simulink model "b_2x_8a_r308d"  (Simulink 6.2)
settings: Solver=ode45  StartTime=0.0  StopTime=1030.0  RelTol=1e-3
undefined symbols (not defined in the file): ant_bits, BEE2_usr, blockCountBits, blockRowBits, cmult_4bit_em
libraries: xbsIndex_r3 x3300, xps_library x102, casper_library x97
(part 14 of 22)

== system b_2x_8a_r308d/win_x_engine1/auto_tap/dual_pol_cmac/cmac1 ==
  a+bi : Inport  Port=1  LatchInput=off
  c+di : Inport  Port=2  LatchInput=off
  acc_in : Inport  Port=3  LatchInput=off
  sync : Inport  Port=4  LatchInput=off
  valid_in : Inport  Port=5  LatchInput=off
  Constant1 : xbsIndex_r3/Constant  const=0  equ=P=C  arith_type=Unsigned  n_bits=bit_growth  bin_pt=0  opselect=C  inp2=PCIN>>17  opr=+  inp1=P  carry=CIN  iostate=0  explicit_period=off  period=1  dbl_ovrd=off
  Constant2 : xbsIndex_r3/Constant  const=0  equ=P=C  arith_type=Unsigned  n_bits=1  bin_pt=0  opselect=C  inp2=PCIN>>17  opr=+  inp1=P  carry=CIN  iostate=0  explicit_period=off  period=1  dbl_ovrd=off
  Counter : xbsIndex_r3/Counter  cnt_type=Count Limited  n_bits=bit_growth  bin_pt=0  arith_type=Unsigned  start_count=0  cnt_to=acc_len - 1  cnt_by_val=1  operation=Up  explicit_period=off  period=1  load_pin=off  rst=on  en=off  dbl_ovrd=off  show_param=off  use_rpm=on  gen_core=off
      settings: xl_area=[0, 0, 0, 0, 0, 0, 0]
  Delay : xbsIndex_r3/Delay  latency=add_latency + mult_latency - 1  reg_retiming=off  explicit_period=off  period=1  en=off  accept_only_valid=off  init_zero=on  dbl_ovrd=off  show_param=off
      settings: xl_area=[0, 0, 0, 0, 0, 0, 0]
  Relational : xbsIndex_r3/Relational  mode=a=b  latency=1  explicit_period=off  period=1  en=off  dbl_ovrd=off  show_param=off
      settings: xl_area=[0, 0, 0, 0, 0, 0, 0]
  Terminator : Terminator
  acc : Subsystem
  acc1 : Subsystem
  c_to_ri : Subsystem
  c_to_ri1 : Subsystem
  c_to_ri2 : Subsystem
  cmult* : Subsystem  BlockChoice=cmult_4bit_em*
      link override cmult_4bit_br*: mult_latency=mult_latency  add_latency=add_latency
      link override cmult_4bit_em*: mult_latency=mult_latency  add_latency=add_latency
      link override cmult_4bit_sl*: mult_latency=mult_latency  add_latency=add_latency
      settings: AttributesFormatString=%<BlockChoice>  TemplateBlock=casper_library/Multipliers/cmult*  MemberBlocks=cmult_4bit_br*,cmult_4bit_em*,cmult_4bit_sl*
      mask Type: cmult*
  ri_to_c : Subsystem
  acc_out : Outport
  valid_out : Outport  Port=2
  wires:
  valid_in/1 -> acc1/4(valid_in)
  acc1/2(valid_out) -> valid_out/1
  acc/2(valid_out) -> Terminator/1
  Constant2/1 -> acc/4(valid_in)
  Delay/1 -> Counter/1
  sync/1 -> Delay/1
  Constant1/1 -> Relational/2
  Counter/1 -> Relational/1
  Relational/1 -> acc1/1(rst), acc/1(rst)
  c_to_ri2/2(Out2) -> acc1/3(acc_in)
  c_to_ri2/1(Out1) -> acc/3(acc_in)
  ri_to_c/1(Out1) -> acc_out/1
  acc1/1(acc_out) -> ri_to_c/2(In2)
  acc/1(acc_out) -> ri_to_c/1(In1)
  acc_in/1 -> c_to_ri2/1(In1)
  c_to_ri1/2(Out2) -> cmult*/4(d)
  c_to_ri1/1(Out1) -> cmult*/3(c)
  c+di/1 -> c_to_ri1/1(In1)
  c_to_ri/2(Out2) -> cmult*/2(b)
  c_to_ri/1(Out1) -> cmult*/1(a)
  a+bi/1 -> c_to_ri/1(In1)
  cmult*/2(imag) -> acc1/2(din)
  cmult*/1(real) -> acc/2(din)

== system b_2x_8a_r308d/win_x_engine1/auto_tap/dual_pol_cmac/cmac2 ==
  a+bi : Inport  Port=1  LatchInput=off
  c+di : Inport  Port=2  LatchInput=off
  acc_in : Inport  Port=3  LatchInput=off
  sync : Inport  Port=4  LatchInput=off
  valid_in : Inport  Port=5  LatchInput=off
  Constant1 : xbsIndex_r3/Constant  const=0  equ=P=C  arith_type=Unsigned  n_bits=bit_growth  bin_pt=0  opselect=C  inp2=PCIN>>17  opr=+  inp1=P  carry=CIN  iostate=0  explicit_period=off  period=1  dbl_ovrd=off
  Constant2 : xbsIndex_r3/Constant  const=0  equ=P=C  arith_type=Unsigned  n_bits=1  bin_pt=0  opselect=C  inp2=PCIN>>17  opr=+  inp1=P  carry=CIN  iostate=0  explicit_period=off  period=1  dbl_ovrd=off
  Counter : xbsIndex_r3/Counter  cnt_type=Count Limited  n_bits=bit_growth  bin_pt=0  arith_type=Unsigned  start_count=0  cnt_to=acc_len - 1  cnt_by_val=1  operation=Up  explicit_period=off  period=1  load_pin=off  rst=on  en=off  dbl_ovrd=off  show_param=off  use_rpm=on  gen_core=off
      settings: xl_area=[0, 0, 0, 0, 0, 0, 0]
  Delay : xbsIndex_r3/Delay  latency=add_latency + mult_latency - 1  reg_retiming=off  explicit_period=off  period=1  en=off  accept_only_valid=off  init_zero=on  dbl_ovrd=off  show_param=off
      settings: xl_area=[0, 0, 0, 0, 0, 0, 0]
  Relational : xbsIndex_r3/Relational  mode=a=b  latency=1  explicit_period=off  period=1  en=off  dbl_ovrd=off  show_param=off
      settings: xl_area=[0, 0, 0, 0, 0, 0, 0]
  Terminator : Terminator
  acc : Subsystem
  acc1 : Subsystem
  c_to_ri : Subsystem
  c_to_ri1 : Subsystem
  c_to_ri2 : Subsystem
  cmult* : Subsystem  BlockChoice=cmult_4bit_em*
      link override cmult_4bit_br*: mult_latency=mult_latency  add_latency=add_latency
      link override cmult_4bit_em*: mult_latency=mult_latency  add_latency=add_latency
      link override cmult_4bit_sl*: mult_latency=mult_latency  add_latency=add_latency
      settings: AttributesFormatString=%<BlockChoice>  TemplateBlock=casper_library/Multipliers/cmult*  MemberBlocks=cmult_4bit_br*,cmult_4bit_em*,cmult_4bit_sl*
      mask Type: cmult*
  ri_to_c : Subsystem
  acc_out : Outport
  valid_out : Outport  Port=2
  wires:
  cmult*/1(real) -> acc/2(din)
  cmult*/2(imag) -> acc1/2(din)
  a+bi/1 -> c_to_ri/1(In1)
  c_to_ri/1(Out1) -> cmult*/1(a)
  c_to_ri/2(Out2) -> cmult*/2(b)
  c+di/1 -> c_to_ri1/1(In1)
  c_to_ri1/1(Out1) -> cmult*/3(c)
  c_to_ri1/2(Out2) -> cmult*/4(d)
  acc_in/1 -> c_to_ri2/1(In1)
  acc/1(acc_out) -> ri_to_c/1(In1)
  acc1/1(acc_out) -> ri_to_c/2(In2)
  ri_to_c/1(Out1) -> acc_out/1
  c_to_ri2/1(Out1) -> acc/3(acc_in)
  c_to_ri2/2(Out2) -> acc1/3(acc_in)
  Relational/1 -> acc/1(rst), acc1/1(rst)
  Counter/1 -> Relational/1
  Constant1/1 -> Relational/2
  sync/1 -> Delay/1
  Delay/1 -> Counter/1
  Constant2/1 -> acc/4(valid_in)
  acc/2(valid_out) -> Terminator/1
  acc1/2(valid_out) -> valid_out/1
  valid_in/1 -> acc1/4(valid_in)

== system b_2x_8a_r308d/win_x_engine1/auto_tap/dual_pol_cmac/cmac3 ==
  a+bi : Inport  Port=1  LatchInput=off
  c+di : Inport  Port=2  LatchInput=off
  acc_in : Inport  Port=3  LatchInput=off
  sync : Inport  Port=4  LatchInput=off
  valid_in : Inport  Port=5  LatchInput=off
  Constant1 : xbsIndex_r3/Constant  const=0  equ=P=C  arith_type=Unsigned  n_bits=bit_growth  bin_pt=0  opselect=C  inp2=PCIN>>17  opr=+  inp1=P  carry=CIN  iostate=0  explicit_period=off  period=1  dbl_ovrd=off
  Constant2 : xbsIndex_r3/Constant  const=0  equ=P=C  arith_type=Unsigned  n_bits=1  bin_pt=0  opselect=C  inp2=PCIN>>17  opr=+  inp1=P  carry=CIN  iostate=0  explicit_period=off  period=1  dbl_ovrd=off
  Counter : xbsIndex_r3/Counter  cnt_type=Count Limited  n_bits=bit_growth  bin_pt=0  arith_type=Unsigned  start_count=0  cnt_to=acc_len - 1  cnt_by_val=1  operation=Up  explicit_period=off  period=1  load_pin=off  rst=on  en=off  dbl_ovrd=off  show_param=off  use_rpm=on  gen_core=off
      settings: xl_area=[0, 0, 0, 0, 0, 0, 0]
  Delay : xbsIndex_r3/Delay  latency=add_latency + mult_latency - 1  reg_retiming=off  explicit_period=off  period=1  en=off  accept_only_valid=off  init_zero=on  dbl_ovrd=off  show_param=off
      settings: xl_area=[0, 0, 0, 0, 0, 0, 0]
  Relational : xbsIndex_r3/Relational  mode=a=b  latency=1  explicit_period=off  period=1  en=off  dbl_ovrd=off  show_param=off
      settings: xl_area=[0, 0, 0, 0, 0, 0, 0]
  Terminator : Terminator
  acc : Subsystem
  acc1 : Subsystem
  c_to_ri : Subsystem
  c_to_ri1 : Subsystem
  c_to_ri2 : Subsystem
  cmult* : Subsystem  BlockChoice=cmult_4bit_em*
      link override cmult_4bit_br*: mult_latency=mult_latency  add_latency=add_latency
      link override cmult_4bit_em*: mult_latency=mult_latency  add_latency=add_latency
      link override cmult_4bit_sl*: mult_latency=mult_latency  add_latency=add_latency
      settings: AttributesFormatString=%<BlockChoice>  TemplateBlock=casper_library/Multipliers/cmult*  MemberBlocks=cmult_4bit_br*,cmult_4bit_em*,cmult_4bit_sl*
      mask Type: cmult*
  ri_to_c : Subsystem
  acc_out : Outport
  valid_out : Outport  Port=2
  wires:
  cmult*/1(real) -> acc/2(din)
  cmult*/2(imag) -> acc1/2(din)
  a+bi/1 -> c_to_ri/1(In1)
  c_to_ri/1(Out1) -> cmult*/1(a)
  c_to_ri/2(Out2) -> cmult*/2(b)
  c+di/1 -> c_to_ri1/1(In1)
  c_to_ri1/1(Out1) -> cmult*/3(c)
  c_to_ri1/2(Out2) -> cmult*/4(d)
  acc_in/1 -> c_to_ri2/1(In1)
  acc/1(acc_out) -> ri_to_c/1(In1)
  acc1/1(acc_out) -> ri_to_c/2(In2)
  ri_to_c/1(Out1) -> acc_out/1
  c_to_ri2/1(Out1) -> acc/3(acc_in)
  c_to_ri2/2(Out2) -> acc1/3(acc_in)
  Relational/1 -> acc/1(rst), acc1/1(rst)
  Counter/1 -> Relational/1
  Constant1/1 -> Relational/2
  sync/1 -> Delay/1
  Delay/1 -> Counter/1
  Constant2/1 -> acc/4(valid_in)
  acc/2(valid_out) -> Terminator/1
  acc1/2(valid_out) -> valid_out/1
  valid_in/1 -> acc1/4(valid_in)

== system b_2x_8a_r308d/win_x_engine1/auto_tap/dual_pol_cmac/cmac4 ==
  a+bi : Inport  Port=1  LatchInput=off
  c+di : Inport  Port=2  LatchInput=off
  acc_in : Inport  Port=3  LatchInput=off
  sync : Inport  Port=4  LatchInput=off
  valid_in : Inport  Port=5  LatchInput=off
  Constant1 : xbsIndex_r3/Constant  const=0  equ=P=C  arith_type=Unsigned  n_bits=bit_growth  bin_pt=0  opselect=C  inp2=PCIN>>17  opr=+  inp1=P  carry=CIN  iostate=0  explicit_period=off  period=1  dbl_ovrd=off
  Constant2 : xbsIndex_r3/Constant  const=0  equ=P=C  arith_type=Unsigned  n_bits=1  bin_pt=0  opselect=C  inp2=PCIN>>17  opr=+  inp1=P  carry=CIN  iostate=0  explicit_period=off  period=1  dbl_ovrd=off
  Counter : xbsIndex_r3/Counter  cnt_type=Count Limited  n_bits=bit_growth  bin_pt=0  arith_type=Unsigned  start_count=0  cnt_to=acc_len - 1  cnt_by_val=1  operation=Up  explicit_period=off  period=1  load_pin=off  rst=on  en=off  dbl_ovrd=off  show_param=off  use_rpm=on  gen_core=off
      settings: xl_area=[0, 0, 0, 0, 0, 0, 0]
  Delay : xbsIndex_r3/Delay  latency=add_latency + mult_latency - 1  reg_retiming=off  explicit_period=off  period=1  en=off  accept_only_valid=off  init_zero=on  dbl_ovrd=off  show_param=off
      settings: xl_area=[0, 0, 0, 0, 0, 0, 0]
  Relational : xbsIndex_r3/Relational  mode=a=b  latency=1  explicit_period=off  period=1  en=off  dbl_ovrd=off  show_param=off
      settings: xl_area=[0, 0, 0, 0, 0, 0, 0]
  Terminator : Terminator
  acc : Subsystem
  acc1 : Subsystem
  c_to_ri : Subsystem
  c_to_ri1 : Subsystem
  c_to_ri2 : Subsystem
  cmult* : Subsystem  BlockChoice=cmult_4bit_em*
      link override cmult_4bit_br*: mult_latency=mult_latency  add_latency=add_latency
      link override cmult_4bit_em*: mult_latency=mult_latency  add_latency=add_latency
      link override cmult_4bit_sl*: mult_latency=mult_latency  add_latency=add_latency
      settings: AttributesFormatString=%<BlockChoice>  TemplateBlock=casper_library/Multipliers/cmult*  MemberBlocks=cmult_4bit_br*,cmult_4bit_em*,cmult_4bit_sl*
      mask Type: cmult*
  ri_to_c : Subsystem
  acc_out : Outport
  valid_out : Outport  Port=2
  wires:
  cmult*/1(real) -> acc/2(din)
  cmult*/2(imag) -> acc1/2(din)
  a+bi/1 -> c_to_ri/1(In1)
  c_to_ri/1(Out1) -> cmult*/1(a)
  c_to_ri/2(Out2) -> cmult*/2(b)
  c+di/1 -> c_to_ri1/1(In1)
  c_to_ri1/1(Out1) -> cmult*/3(c)
  c_to_ri1/2(Out2) -> cmult*/4(d)
  acc_in/1 -> c_to_ri2/1(In1)
  acc/1(acc_out) -> ri_to_c/1(In1)
  acc1/1(acc_out) -> ri_to_c/2(In2)
  ri_to_c/1(Out1) -> acc_out/1
  c_to_ri2/1(Out1) -> acc/3(acc_in)
  c_to_ri2/2(Out2) -> acc1/3(acc_in)
  Relational/1 -> acc/1(rst), acc1/1(rst)
  Counter/1 -> Relational/1
  Constant1/1 -> Relational/2
  sync/1 -> Delay/1
  Delay/1 -> Counter/1
  Constant2/1 -> acc/4(valid_in)
  acc/2(valid_out) -> Terminator/1
  acc1/2(valid_out) -> valid_out/1
  valid_in/1 -> acc1/4(valid_in)

== system b_2x_8a_r308d/win_x_engine1/baseline_tap2/dual_pol_cmac/cmac1 ==
  a+bi : Inport  Port=1  LatchInput=off
  c+di : Inport  Port=2  LatchInput=off
  acc_in : Inport  Port=3  LatchInput=off
  sync : Inport  Port=4  LatchInput=off
  valid_in : Inport  Port=5  LatchInput=off
  Constant1 : xbsIndex_r3/Constant  const=0  equ=P=C  arith_type=Unsigned  n_bits=bit_growth  bin_pt=0  opselect=C  inp2=PCIN>>17  opr=+  inp1=P  carry=CIN  iostate=0  explicit_period=off  period=1  dbl_ovrd=off
  Constant2 : xbsIndex_r3/Constant  const=0  equ=P=C  arith_type=Unsigned  n_bits=1  bin_pt=0  opselect=C  inp2=PCIN>>17  opr=+  inp1=P  carry=CIN  iostate=0  explicit_period=off  period=1  dbl_ovrd=off
  Counter : xbsIndex_r3/Counter  cnt_type=Count Limited  n_bits=bit_growth  bin_pt=0  arith_type=Unsigned  start_count=0  cnt_to=acc_len - 1  cnt_by_val=1  operation=Up  explicit_period=off  period=1  load_pin=off  rst=on  en=off  dbl_ovrd=off  show_param=off  use_rpm=on  gen_core=off
      settings: xl_area=[0, 0, 0, 0, 0, 0, 0]
  Delay : xbsIndex_r3/Delay  latency=add_latency + mult_latency - 1  reg_retiming=off  explicit_period=off  period=1  en=off  accept_only_valid=off  init_zero=on  dbl_ovrd=off  show_param=off
      settings: xl_area=[0, 0, 0, 0, 0, 0, 0]
  Relational : xbsIndex_r3/Relational  mode=a=b  latency=1  explicit_period=off  period=1  en=off  dbl_ovrd=off  show_param=off
      settings: xl_area=[0, 0, 0, 0, 0, 0, 0]
  Terminator : Terminator
  acc : Subsystem
  acc1 : Subsystem
  c_to_ri : Subsystem
  c_to_ri1 : Subsystem
  c_to_ri2 : Subsystem
  cmult* : Subsystem  BlockChoice=cmult_4bit_em*
      link override cmult_4bit_br*: mult_latency=mult_latency  add_latency=add_latency
      link override cmult_4bit_em*: mult_latency=mult_latency  add_latency=add_latency
      link override cmult_4bit_sl*: mult_latency=mult_latency  add_latency=add_latency
      settings: AttributesFormatString=%<BlockChoice>  TemplateBlock=casper_library/Multipliers/cmult*  MemberBlocks=cmult_4bit_br*,cmult_4bit_em*,cmult_4bit_sl*
      mask Type: cmult*
  ri_to_c : Subsystem
  acc_out : Outport
  valid_out : Outport  Port=2
  wires:
  cmult*/1(real) -> acc/2(din)
  cmult*/2(imag) -> acc1/2(din)
  a+bi/1 -> c_to_ri/1(In1)
  c_to_ri/1(Out1) -> cmult*/1(a)
  c_to_ri/2(Out2) -> cmult*/2(b)
  c+di/1 -> c_to_ri1/1(In1)
  c_to_ri1/1(Out1) -> cmult*/3(c)
  c_to_ri1/2(Out2) -> cmult*/4(d)
  acc_in/1 -> c_to_ri2/1(In1)
  acc/1(acc_out) -> ri_to_c/1(In1)
  acc1/1(acc_out) -> ri_to_c/2(In2)
  ri_to_c/1(Out1) -> acc_out/1
  c_to_ri2/1(Out1) -> acc/3(acc_in)
  c_to_ri2/2(Out2) -> acc1/3(acc_in)
  Relational/1 -> acc/1(rst), acc1/1(rst)
  Counter/1 -> Relational/1
  Constant1/1 -> Relational/2
  sync/1 -> Delay/1
  Delay/1 -> Counter/1
  Constant2/1 -> acc/4(valid_in)
  acc/2(valid_out) -> Terminator/1
  acc1/2(valid_out) -> valid_out/1
  valid_in/1 -> acc1/4(valid_in)

== system b_2x_8a_r308d/win_x_engine1/baseline_tap2/dual_pol_cmac/cmac2 ==
  a+bi : Inport  Port=1  LatchInput=off
  c+di : Inport  Port=2  LatchInput=off
  acc_in : Inport  Port=3  LatchInput=off
  sync : Inport  Port=4  LatchInput=off
  valid_in : Inport  Port=5  LatchInput=off
  Constant1 : xbsIndex_r3/Constant  const=0  equ=P=C  arith_type=Unsigned  n_bits=bit_growth  bin_pt=0  opselect=C  inp2=PCIN>>17  opr=+  inp1=P  carry=CIN  iostate=0  explicit_period=off  period=1  dbl_ovrd=off
  Constant2 : xbsIndex_r3/Constant  const=0  equ=P=C  arith_type=Unsigned  n_bits=1  bin_pt=0  opselect=C  inp2=PCIN>>17  opr=+  inp1=P  carry=CIN  iostate=0  explicit_period=off  period=1  dbl_ovrd=off
  Counter : xbsIndex_r3/Counter  cnt_type=Count Limited  n_bits=bit_growth  bin_pt=0  arith_type=Unsigned  start_count=0  cnt_to=acc_len - 1  cnt_by_val=1  operation=Up  explicit_period=off  period=1  load_pin=off  rst=on  en=off  dbl_ovrd=off  show_param=off  use_rpm=on  gen_core=off
      settings: xl_area=[0, 0, 0, 0, 0, 0, 0]
  Delay : xbsIndex_r3/Delay  latency=add_latency + mult_latency - 1  reg_retiming=off  explicit_period=off  period=1  en=off  accept_only_valid=off  init_zero=on  dbl_ovrd=off  show_param=off
      settings: xl_area=[0, 0, 0, 0, 0, 0, 0]
  Relational : xbsIndex_r3/Relational  mode=a=b  latency=1  explicit_period=off  period=1  en=off  dbl_ovrd=off  show_param=off
      settings: xl_area=[0, 0, 0, 0, 0, 0, 0]
  Terminator : Terminator
  acc : Subsystem
  acc1 : Subsystem
  c_to_ri : Subsystem
  c_to_ri1 : Subsystem
  c_to_ri2 : Subsystem
  cmult* : Subsystem  BlockChoice=cmult_4bit_em*
      link override cmult_4bit_br*: mult_latency=mult_latency  add_latency=add_latency
      link override cmult_4bit_em*: mult_latency=mult_latency  add_latency=add_latency
      link override cmult_4bit_sl*: mult_latency=mult_latency  add_latency=add_latency
      settings: AttributesFormatString=%<BlockChoice>  TemplateBlock=casper_library/Multipliers/cmult*  MemberBlocks=cmult_4bit_br*,cmult_4bit_em*,cmult_4bit_sl*
      mask Type: cmult*
  ri_to_c : Subsystem
  acc_out : Outport
  valid_out : Outport  Port=2
  wires:
  valid_in/1 -> acc1/4(valid_in)
  acc1/2(valid_out) -> valid_out/1
  acc/2(valid_out) -> Terminator/1
  Constant2/1 -> acc/4(valid_in)
  Delay/1 -> Counter/1
  sync/1 -> Delay/1
  Constant1/1 -> Relational/2
  Counter/1 -> Relational/1
  Relational/1 -> acc1/1(rst), acc/1(rst)
  c_to_ri2/2(Out2) -> acc1/3(acc_in)
  c_to_ri2/1(Out1) -> acc/3(acc_in)
  ri_to_c/1(Out1) -> acc_out/1
  acc1/1(acc_out) -> ri_to_c/2(In2)
  acc/1(acc_out) -> ri_to_c/1(In1)
  acc_in/1 -> c_to_ri2/1(In1)
  c_to_ri1/2(Out2) -> cmult*/4(d)
  c_to_ri1/1(Out1) -> cmult*/3(c)
  c+di/1 -> c_to_ri1/1(In1)
  c_to_ri/2(Out2) -> cmult*/2(b)
  c_to_ri/1(Out1) -> cmult*/1(a)
  a+bi/1 -> c_to_ri/1(In1)
  cmult*/2(imag) -> acc1/2(din)
  cmult*/1(real) -> acc/2(din)

== system b_2x_8a_r308d/win_x_engine1/baseline_tap2/dual_pol_cmac/cmac3 ==
  a+bi : Inport  Port=1  LatchInput=off
  c+di : Inport  Port=2  LatchInput=off
  acc_in : Inport  Port=3  LatchInput=off
  sync : Inport  Port=4  LatchInput=off
  valid_in : Inport  Port=5  LatchInput=off
  Constant1 : xbsIndex_r3/Constant  const=0  equ=P=C  arith_type=Unsigned  n_bits=bit_growth  bin_pt=0  opselect=C  inp2=PCIN>>17  opr=+  inp1=P  carry=CIN  iostate=0  explicit_period=off  period=1  dbl_ovrd=off
  Constant2 : xbsIndex_r3/Constant  const=0  equ=P=C  arith_type=Unsigned  n_bits=1  bin_pt=0  opselect=C  inp2=PCIN>>17  opr=+  inp1=P  carry=CIN  iostate=0  explicit_period=off  period=1  dbl_ovrd=off
  Counter : xbsIndex_r3/Counter  cnt_type=Count Limited  n_bits=bit_growth  bin_pt=0  arith_type=Unsigned  start_count=0  cnt_to=acc_len - 1  cnt_by_val=1  operation=Up  explicit_period=off  period=1  load_pin=off  rst=on  en=off  dbl_ovrd=off  show_param=off  use_rpm=on  gen_core=off
      settings: xl_area=[0, 0, 0, 0, 0, 0, 0]
  Delay : xbsIndex_r3/Delay  latency=add_latency + mult_latency - 1  reg_retiming=off  explicit_period=off  period=1  en=off  accept_only_valid=off  init_zero=on  dbl_ovrd=off  show_param=off
      settings: xl_area=[0, 0, 0, 0, 0, 0, 0]
  Relational : xbsIndex_r3/Relational  mode=a=b  latency=1  explicit_period=off  period=1  en=off  dbl_ovrd=off  show_param=off
      settings: xl_area=[0, 0, 0, 0, 0, 0, 0]
  Terminator : Terminator
  acc : Subsystem
  acc1 : Subsystem
  c_to_ri : Subsystem
  c_to_ri1 : Subsystem
  c_to_ri2 : Subsystem
  cmult* : Subsystem  BlockChoice=cmult_4bit_em*
      link override cmult_4bit_br*: mult_latency=mult_latency  add_latency=add_latency
      link override cmult_4bit_em*: mult_latency=mult_latency  add_latency=add_latency
      link override cmult_4bit_sl*: mult_latency=mult_latency  add_latency=add_latency
      settings: AttributesFormatString=%<BlockChoice>  TemplateBlock=casper_library/Multipliers/cmult*  MemberBlocks=cmult_4bit_br*,cmult_4bit_em*,cmult_4bit_sl*
      mask Type: cmult*
  ri_to_c : Subsystem
  acc_out : Outport
  valid_out : Outport  Port=2
  wires:
  valid_in/1 -> acc1/4(valid_in)
  acc1/2(valid_out) -> valid_out/1
  acc/2(valid_out) -> Terminator/1
  Constant2/1 -> acc/4(valid_in)
  Delay/1 -> Counter/1
  sync/1 -> Delay/1
  Constant1/1 -> Relational/2
  Counter/1 -> Relational/1
  Relational/1 -> acc1/1(rst), acc/1(rst)
  c_to_ri2/2(Out2) -> acc1/3(acc_in)
  c_to_ri2/1(Out1) -> acc/3(acc_in)
  ri_to_c/1(Out1) -> acc_out/1
  acc1/1(acc_out) -> ri_to_c/2(In2)
  acc/1(acc_out) -> ri_to_c/1(In1)
  acc_in/1 -> c_to_ri2/1(In1)
  c_to_ri1/2(Out2) -> cmult*/4(d)
  c_to_ri1/1(Out1) -> cmult*/3(c)
  c+di/1 -> c_to_ri1/1(In1)
  c_to_ri/2(Out2) -> cmult*/2(b)
  c_to_ri/1(Out1) -> cmult*/1(a)
  a+bi/1 -> c_to_ri/1(In1)
  cmult*/2(imag) -> acc1/2(din)
  cmult*/1(real) -> acc/2(din)

== system b_2x_8a_r308d/win_x_engine1/baseline_tap2/dual_pol_cmac/cmac4 ==
  a+bi : Inport  Port=1  LatchInput=off
  c+di : Inport  Port=2  LatchInput=off
  acc_in : Inport  Port=3  LatchInput=off
  sync : Inport  Port=4  LatchInput=off
  valid_in : Inport  Port=5  LatchInput=off
  Constant1 : xbsIndex_r3/Constant  const=0  equ=P=C  arith_type=Unsigned  n_bits=bit_growth  bin_pt=0  opselect=C  inp2=PCIN>>17  opr=+  inp1=P  carry=CIN  iostate=0  explicit_period=off  period=1  dbl_ovrd=off
  Constant2 : xbsIndex_r3/Constant  const=0  equ=P=C  arith_type=Unsigned  n_bits=1  bin_pt=0  opselect=C  inp2=PCIN>>17  opr=+  inp1=P  carry=CIN  iostate=0  explicit_period=off  period=1  dbl_ovrd=off
  Counter : xbsIndex_r3/Counter  cnt_type=Count Limited  n_bits=bit_growth  bin_pt=0  arith_type=Unsigned  start_count=0  cnt_to=acc_len - 1  cnt_by_val=1  operation=Up  explicit_period=off  period=1  load_pin=off  rst=on  en=off  dbl_ovrd=off  show_param=off  use_rpm=on  gen_core=off
      settings: xl_area=[0, 0, 0, 0, 0, 0, 0]
  Delay : xbsIndex_r3/Delay  latency=add_latency + mult_latency - 1  reg_retiming=off  explicit_period=off  period=1  en=off  accept_only_valid=off  init_zero=on  dbl_ovrd=off  show_param=off
      settings: xl_area=[0, 0, 0, 0, 0, 0, 0]
  Relational : xbsIndex_r3/Relational  mode=a=b  latency=1  explicit_period=off  period=1  en=off  dbl_ovrd=off  show_param=off
      settings: xl_area=[0, 0, 0, 0, 0, 0, 0]
  Terminator : Terminator
  acc : Subsystem
  acc1 : Subsystem
  c_to_ri : Subsystem
  c_to_ri1 : Subsystem
  c_to_ri2 : Subsystem
  cmult* : Subsystem  BlockChoice=cmult_4bit_em*
      link override cmult_4bit_br*: mult_latency=mult_latency  add_latency=add_latency
      link override cmult_4bit_em*: mult_latency=mult_latency  add_latency=add_latency
      link override cmult_4bit_sl*: mult_latency=mult_latency  add_latency=add_latency
      settings: AttributesFormatString=%<BlockChoice>  TemplateBlock=casper_library/Multipliers/cmult*  MemberBlocks=cmult_4bit_br*,cmult_4bit_em*,cmult_4bit_sl*
      mask Type: cmult*
  ri_to_c : Subsystem
  acc_out : Outport
  valid_out : Outport  Port=2
  wires:
  valid_in/1 -> acc1/4(valid_in)
  acc1/2(valid_out) -> valid_out/1
  acc/2(valid_out) -> Terminator/1
  Constant2/1 -> acc/4(valid_in)
  Delay/1 -> Counter/1
  sync/1 -> Delay/1
  Constant1/1 -> Relational/2
  Counter/1 -> Relational/1
  Relational/1 -> acc1/1(rst), acc/1(rst)
  c_to_ri2/2(Out2) -> acc1/3(acc_in)
  c_to_ri2/1(Out1) -> acc/3(acc_in)
  ri_to_c/1(Out1) -> acc_out/1
  acc1/1(acc_out) -> ri_to_c/2(In2)
  acc/1(acc_out) -> ri_to_c/1(In1)
  acc_in/1 -> c_to_ri2/1(In1)
  c_to_ri1/2(Out2) -> cmult*/4(d)
  c_to_ri1/1(Out1) -> cmult*/3(c)
  c+di/1 -> c_to_ri1/1(In1)
  c_to_ri/2(Out2) -> cmult*/2(b)
  c_to_ri/1(Out1) -> cmult*/1(a)
  a+bi/1 -> c_to_ri/1(In1)
  cmult*/2(imag) -> acc1/2(din)
  cmult*/1(real) -> acc/2(din)

== system b_2x_8a_r308d/win_x_engine1/baseline_tap3/dual_pol_cmac/cmac1 ==
  a+bi : Inport  Port=1  LatchInput=off
  c+di : Inport  Port=2  LatchInput=off
  acc_in : Inport  Port=3  LatchInput=off
  sync : Inport  Port=4  LatchInput=off
  valid_in : Inport  Port=5  LatchInput=off
  Constant1 : xbsIndex_r3/Constant  const=0  equ=P=C  arith_type=Unsigned  n_bits=bit_growth  bin_pt=0  opselect=C  inp2=PCIN>>17  opr=+  inp1=P  carry=CIN  iostate=0  explicit_period=off  period=1  dbl_ovrd=off
  Constant2 : xbsIndex_r3/Constant  const=0  equ=P=C  arith_type=Unsigned  n_bits=1  bin_pt=0  opselect=C  inp2=PCIN>>17  opr=+  inp1=P  carry=CIN  iostate=0  explicit_period=off  period=1  dbl_ovrd=off
  Counter : xbsIndex_r3/Counter  cnt_type=Count Limited  n_bits=bit_growth  bin_pt=0  arith_type=Unsigned  start_count=0  cnt_to=acc_len - 1  cnt_by_val=1  operation=Up  explicit_period=off  period=1  load_pin=off  rst=on  en=off  dbl_ovrd=off  show_param=off  use_rpm=on  gen_core=off
      settings: xl_area=[0, 0, 0, 0, 0, 0, 0]
  Delay : xbsIndex_r3/Delay  latency=add_latency + mult_latency - 1  reg_retiming=off  explicit_period=off  period=1  en=off  accept_only_valid=off  init_zero=on  dbl_ovrd=off  show_param=off
      settings: xl_area=[0, 0, 0, 0, 0, 0, 0]
  Relational : xbsIndex_r3/Relational  mode=a=b  latency=1  explicit_period=off  period=1  en=off  dbl_ovrd=off  show_param=off
      settings: xl_area=[0, 0, 0, 0, 0, 0, 0]
  Terminator : Terminator
  acc : Subsystem
  acc1 : Subsystem
  c_to_ri : Subsystem
  c_to_ri1 : Subsystem
  c_to_ri2 : Subsystem
  cmult* : Subsystem  BlockChoice=cmult_4bit_em*
      link override cmult_4bit_br*: mult_latency=mult_latency  add_latency=add_latency
      link override cmult_4bit_em*: mult_latency=mult_latency  add_latency=add_latency
      link override cmult_4bit_sl*: mult_latency=mult_latency  add_latency=add_latency
      settings: AttributesFormatString=%<BlockChoice>  TemplateBlock=casper_library/Multipliers/cmult*  MemberBlocks=cmult_4bit_br*,cmult_4bit_em*,cmult_4bit_sl*
      mask Type: cmult*
  ri_to_c : Subsystem
  acc_out : Outport
  valid_out : Outport  Port=2
  wires:
  cmult*/1(real) -> acc/2(din)
  cmult*/2(imag) -> acc1/2(din)
  a+bi/1 -> c_to_ri/1(In1)
  c_to_ri/1(Out1) -> cmult*/1(a)
  c_to_ri/2(Out2) -> cmult*/2(b)
  c+di/1 -> c_to_ri1/1(In1)
  c_to_ri1/1(Out1) -> cmult*/3(c)
  c_to_ri1/2(Out2) -> cmult*/4(d)
  acc_in/1 -> c_to_ri2/1(In1)
  acc/1(acc_out) -> ri_to_c/1(In1)
  acc1/1(acc_out) -> ri_to_c/2(In2)
  ri_to_c/1(Out1) -> acc_out/1
  c_to_ri2/1(Out1) -> acc/3(acc_in)
  c_to_ri2/2(Out2) -> acc1/3(acc_in)
  Relational/1 -> acc/1(rst), acc1/1(rst)
  Counter/1 -> Relational/1
  Constant1/1 -> Relational/2
  sync/1 -> Delay/1
  Delay/1 -> Counter/1
  Constant2/1 -> acc/4(valid_in)
  acc/2(valid_out) -> Terminator/1
  acc1/2(valid_out) -> valid_out/1
  valid_in/1 -> acc1/4(valid_in)

== system b_2x_8a_r308d/win_x_engine1/baseline_tap3/dual_pol_cmac/cmac2 ==
  a+bi : Inport  Port=1  LatchInput=off
  c+di : Inport  Port=2  LatchInput=off
  acc_in : Inport  Port=3  LatchInput=off
  sync : Inport  Port=4  LatchInput=off
  valid_in : Inport  Port=5  LatchInput=off
  Constant1 : xbsIndex_r3/Constant  const=0  equ=P=C  arith_type=Unsigned  n_bits=bit_growth  bin_pt=0  opselect=C  inp2=PCIN>>17  opr=+  inp1=P  carry=CIN  iostate=0  explicit_period=off  period=1  dbl_ovrd=off
  Constant2 : xbsIndex_r3/Constant  const=0  equ=P=C  arith_type=Unsigned  n_bits=1  bin_pt=0  opselect=C  inp2=PCIN>>17  opr=+  inp1=P  carry=CIN  iostate=0  explicit_period=off  period=1  dbl_ovrd=off
  Counter : xbsIndex_r3/Counter  cnt_type=Count Limited  n_bits=bit_growth  bin_pt=0  arith_type=Unsigned  start_count=0  cnt_to=acc_len - 1  cnt_by_val=1  operation=Up  explicit_period=off  period=1  load_pin=off  rst=on  en=off  dbl_ovrd=off  show_param=off  use_rpm=on  gen_core=off
      settings: xl_area=[0, 0, 0, 0, 0, 0, 0]
  Delay : xbsIndex_r3/Delay  latency=add_latency + mult_latency - 1  reg_retiming=off  explicit_period=off  period=1  en=off  accept_only_valid=off  init_zero=on  dbl_ovrd=off  show_param=off
      settings: xl_area=[0, 0, 0, 0, 0, 0, 0]
  Relational : xbsIndex_r3/Relational  mode=a=b  latency=1  explicit_period=off  period=1  en=off  dbl_ovrd=off  show_param=off
      settings: xl_area=[0, 0, 0, 0, 0, 0, 0]
  Terminator : Terminator
  acc : Subsystem
  acc1 : Subsystem
  c_to_ri : Subsystem
  c_to_ri1 : Subsystem
  c_to_ri2 : Subsystem
  cmult* : Subsystem  BlockChoice=cmult_4bit_em*
      link override cmult_4bit_br*: mult_latency=mult_latency  add_latency=add_latency
      link override cmult_4bit_em*: mult_latency=mult_latency  add_latency=add_latency
      link override cmult_4bit_sl*: mult_latency=mult_latency  add_latency=add_latency
      settings: AttributesFormatString=%<BlockChoice>  TemplateBlock=casper_library/Multipliers/cmult*  MemberBlocks=cmult_4bit_br*,cmult_4bit_em*,cmult_4bit_sl*
      mask Type: cmult*
  ri_to_c : Subsystem
  acc_out : Outport
  valid_out : Outport  Port=2
  wires:
  valid_in/1 -> acc1/4(valid_in)
  acc1/2(valid_out) -> valid_out/1
  acc/2(valid_out) -> Terminator/1
  Constant2/1 -> acc/4(valid_in)
  Delay/1 -> Counter/1
  sync/1 -> Delay/1
  Constant1/1 -> Relational/2
  Counter/1 -> Relational/1
  Relational/1 -> acc1/1(rst), acc/1(rst)
  c_to_ri2/2(Out2) -> acc1/3(acc_in)
  c_to_ri2/1(Out1) -> acc/3(acc_in)
  ri_to_c/1(Out1) -> acc_out/1
  acc1/1(acc_out) -> ri_to_c/2(In2)
  acc/1(acc_out) -> ri_to_c/1(In1)
  acc_in/1 -> c_to_ri2/1(In1)
  c_to_ri1/2(Out2) -> cmult*/4(d)
  c_to_ri1/1(Out1) -> cmult*/3(c)
  c+di/1 -> c_to_ri1/1(In1)
  c_to_ri/2(Out2) -> cmult*/2(b)
  c_to_ri/1(Out1) -> cmult*/1(a)
  a+bi/1 -> c_to_ri/1(In1)
  cmult*/2(imag) -> acc1/2(din)
  cmult*/1(real) -> acc/2(din)

== system b_2x_8a_r308d/win_x_engine1/baseline_tap3/dual_pol_cmac/cmac3 ==
  a+bi : Inport  Port=1  LatchInput=off
  c+di : Inport  Port=2  LatchInput=off
  acc_in : Inport  Port=3  LatchInput=off
  sync : Inport  Port=4  LatchInput=off
  valid_in : Inport  Port=5  LatchInput=off
  Constant1 : xbsIndex_r3/Constant  const=0  equ=P=C  arith_type=Unsigned  n_bits=bit_growth  bin_pt=0  opselect=C  inp2=PCIN>>17  opr=+  inp1=P  carry=CIN  iostate=0  explicit_period=off  period=1  dbl_ovrd=off
  Constant2 : xbsIndex_r3/Constant  const=0  equ=P=C  arith_type=Unsigned  n_bits=1  bin_pt=0  opselect=C  inp2=PCIN>>17  opr=+  inp1=P  carry=CIN  iostate=0  explicit_period=off  period=1  dbl_ovrd=off
  Counter : xbsIndex_r3/Counter  cnt_type=Count Limited  n_bits=bit_growth  bin_pt=0  arith_type=Unsigned  start_count=0  cnt_to=acc_len - 1  cnt_by_val=1  operation=Up  explicit_period=off  period=1  load_pin=off  rst=on  en=off  dbl_ovrd=off  show_param=off  use_rpm=on  gen_core=off
      settings: xl_area=[0, 0, 0, 0, 0, 0, 0]
  Delay : xbsIndex_r3/Delay  latency=add_latency + mult_latency - 1  reg_retiming=off  explicit_period=off  period=1  en=off  accept_only_valid=off  init_zero=on  dbl_ovrd=off  show_param=off
      settings: xl_area=[0, 0, 0, 0, 0, 0, 0]
  Relational : xbsIndex_r3/Relational  mode=a=b  latency=1  explicit_period=off  period=1  en=off  dbl_ovrd=off  show_param=off
      settings: xl_area=[0, 0, 0, 0, 0, 0, 0]
  Terminator : Terminator
  acc : Subsystem
  acc1 : Subsystem
  c_to_ri : Subsystem
  c_to_ri1 : Subsystem
  c_to_ri2 : Subsystem
  cmult* : Subsystem  BlockChoice=cmult_4bit_em*
      link override cmult_4bit_br*: mult_latency=mult_latency  add_latency=add_latency
      link override cmult_4bit_em*: mult_latency=mult_latency  add_latency=add_latency
      link override cmult_4bit_sl*: mult_latency=mult_latency  add_latency=add_latency
      settings: AttributesFormatString=%<BlockChoice>  TemplateBlock=casper_library/Multipliers/cmult*  MemberBlocks=cmult_4bit_br*,cmult_4bit_em*,cmult_4bit_sl*
      mask Type: cmult*
  ri_to_c : Subsystem
  acc_out : Outport
  valid_out : Outport  Port=2
  wires:
  valid_in/1 -> acc1/4(valid_in)
  acc1/2(valid_out) -> valid_out/1
  acc/2(valid_out) -> Terminator/1
  Constant2/1 -> acc/4(valid_in)
  Delay/1 -> Counter/1
  sync/1 -> Delay/1
  Constant1/1 -> Relational/2
  Counter/1 -> Relational/1
  Relational/1 -> acc1/1(rst), acc/1(rst)
  c_to_ri2/2(Out2) -> acc1/3(acc_in)
  c_to_ri2/1(Out1) -> acc/3(acc_in)
  ri_to_c/1(Out1) -> acc_out/1
  acc1/1(acc_out) -> ri_to_c/2(In2)
  acc/1(acc_out) -> ri_to_c/1(In1)
  acc_in/1 -> c_to_ri2/1(In1)
  c_to_ri1/2(Out2) -> cmult*/4(d)
  c_to_ri1/1(Out1) -> cmult*/3(c)
  c+di/1 -> c_to_ri1/1(In1)
  c_to_ri/2(Out2) -> cmult*/2(b)
  c_to_ri/1(Out1) -> cmult*/1(a)
  a+bi/1 -> c_to_ri/1(In1)
  cmult*/2(imag) -> acc1/2(din)
  cmult*/1(real) -> acc/2(din)

== system b_2x_8a_r308d/win_x_engine1/baseline_tap3/dual_pol_cmac/cmac4 ==
  a+bi : Inport  Port=1  LatchInput=off
  c+di : Inport  Port=2  LatchInput=off
  acc_in : Inport  Port=3  LatchInput=off
  sync : Inport  Port=4  LatchInput=off
  valid_in : Inport  Port=5  LatchInput=off
  Constant1 : xbsIndex_r3/Constant  const=0  equ=P=C  arith_type=Unsigned  n_bits=bit_growth  bin_pt=0  opselect=C  inp2=PCIN>>17  opr=+  inp1=P  carry=CIN  iostate=0  explicit_period=off  period=1  dbl_ovrd=off
  Constant2 : xbsIndex_r3/Constant  const=0  equ=P=C  arith_type=Unsigned  n_bits=1  bin_pt=0  opselect=C  inp2=PCIN>>17  opr=+  inp1=P  carry=CIN  iostate=0  explicit_period=off  period=1  dbl_ovrd=off
  Counter : xbsIndex_r3/Counter  cnt_type=Count Limited  n_bits=bit_growth  bin_pt=0  arith_type=Unsigned  start_count=0  cnt_to=acc_len - 1  cnt_by_val=1  operation=Up  explicit_period=off  period=1  load_pin=off  rst=on  en=off  dbl_ovrd=off  show_param=off  use_rpm=on  gen_core=off
      settings: xl_area=[0, 0, 0, 0, 0, 0, 0]
  Delay : xbsIndex_r3/Delay  latency=add_latency + mult_latency - 1  reg_retiming=off  explicit_period=off  period=1  en=off  accept_only_valid=off  init_zero=on  dbl_ovrd=off  show_param=off
      settings: xl_area=[0, 0, 0, 0, 0, 0, 0]
  Relational : xbsIndex_r3/Relational  mode=a=b  latency=1  explicit_period=off  period=1  en=off  dbl_ovrd=off  show_param=off
      settings: xl_area=[0, 0, 0, 0, 0, 0, 0]
  Terminator : Terminator
  acc : Subsystem
  acc1 : Subsystem
  c_to_ri : Subsystem
  c_to_ri1 : Subsystem
  c_to_ri2 : Subsystem
  cmult* : Subsystem  BlockChoice=cmult_4bit_em*
      link override cmult_4bit_br*: mult_latency=mult_latency  add_latency=add_latency
      link override cmult_4bit_em*: mult_latency=mult_latency  add_latency=add_latency
      link override cmult_4bit_sl*: mult_latency=mult_latency  add_latency=add_latency
      settings: AttributesFormatString=%<BlockChoice>  TemplateBlock=casper_library/Multipliers/cmult*  MemberBlocks=cmult_4bit_br*,cmult_4bit_em*,cmult_4bit_sl*
      mask Type: cmult*
  ri_to_c : Subsystem
  acc_out : Outport
  valid_out : Outport  Port=2
  wires:
  valid_in/1 -> acc1/4(valid_in)
  acc1/2(valid_out) -> valid_out/1
  acc/2(valid_out) -> Terminator/1
  Constant2/1 -> acc/4(valid_in)
  Delay/1 -> Counter/1
  sync/1 -> Delay/1
  Constant1/1 -> Relational/2
  Counter/1 -> Relational/1
  Relational/1 -> acc1/1(rst), acc/1(rst)
  c_to_ri2/2(Out2) -> acc1/3(acc_in)
  c_to_ri2/1(Out1) -> acc/3(acc_in)
  ri_to_c/1(Out1) -> acc_out/1
  acc1/1(acc_out) -> ri_to_c/2(In2)
  acc/1(acc_out) -> ri_to_c/1(In1)
  acc_in/1 -> c_to_ri2/1(In1)
  c_to_ri1/2(Out2) -> cmult*/4(d)
  c_to_ri1/1(Out1) -> cmult*/3(c)
  c+di/1 -> c_to_ri1/1(In1)
  c_to_ri/2(Out2) -> cmult*/2(b)
  c_to_ri/1(Out1) -> cmult*/1(a)
  a+bi/1 -> c_to_ri/1(In1)
  cmult*/2(imag) -> acc1/2(din)
  cmult*/1(real) -> acc/2(din)

== system b_2x_8a_r308d/win_x_engine1/baseline_tap4/dual_pol_cmac/cmac1 ==
  a+bi : Inport  Port=1  LatchInput=off
  c+di : Inport  Port=2  LatchInput=off
  acc_in : Inport  Port=3  LatchInput=off
  sync : Inport  Port=4  LatchInput=off
  valid_in : Inport  Port=5  LatchInput=off
  Constant1 : xbsIndex_r3/Constant  const=0  equ=P=C  arith_type=Unsigned  n_bits=bit_growth  bin_pt=0  opselect=C  inp2=PCIN>>17  opr=+  inp1=P  carry=CIN  iostate=0  explicit_period=off  period=1  dbl_ovrd=off
  Constant2 : xbsIndex_r3/Constant  const=0  equ=P=C  arith_type=Unsigned  n_bits=1  bin_pt=0  opselect=C  inp2=PCIN>>17  opr=+  inp1=P  carry=CIN  iostate=0  explicit_period=off  period=1  dbl_ovrd=off
  Counter : xbsIndex_r3/Counter  cnt_type=Count Limited  n_bits=bit_growth  bin_pt=0  arith_type=Unsigned  start_count=0  cnt_to=acc_len - 1  cnt_by_val=1  operation=Up  explicit_period=off  period=1  load_pin=off  rst=on  en=off  dbl_ovrd=off  show_param=off  use_rpm=on  gen_core=off
      settings: xl_area=[0, 0, 0, 0, 0, 0, 0]
  Delay : xbsIndex_r3/Delay  latency=add_latency + mult_latency - 1  reg_retiming=off  explicit_period=off  period=1  en=off  accept_only_valid=off  init_zero=on  dbl_ovrd=off  show_param=off
      settings: xl_area=[0, 0, 0, 0, 0, 0, 0]
  Relational : xbsIndex_r3/Relational  mode=a=b  latency=1  explicit_period=off  period=1  en=off  dbl_ovrd=off  show_param=off
      settings: xl_area=[0, 0, 0, 0, 0, 0, 0]
  Terminator : Terminator
  acc : Subsystem
  acc1 : Subsystem
  c_to_ri : Subsystem
  c_to_ri1 : Subsystem
  c_to_ri2 : Subsystem
  cmult* : Subsystem  BlockChoice=cmult_4bit_em*
      link override cmult_4bit_br*: mult_latency=mult_latency  add_latency=add_latency
      link override cmult_4bit_em*: mult_latency=mult_latency  add_latency=add_latency
      link override cmult_4bit_sl*: mult_latency=mult_latency  add_latency=add_latency
      settings: AttributesFormatString=%<BlockChoice>  TemplateBlock=casper_library/Multipliers/cmult*  MemberBlocks=cmult_4bit_br*,cmult_4bit_em*,cmult_4bit_sl*
      mask Type: cmult*
  ri_to_c : Subsystem
  acc_out : Outport
  valid_out : Outport  Port=2
  wires:
  cmult*/1(real) -> acc/2(din)
  cmult*/2(imag) -> acc1/2(din)
  a+bi/1 -> c_to_ri/1(In1)
  c_to_ri/1(Out1) -> cmult*/1(a)
  c_to_ri/2(Out2) -> cmult*/2(b)
  c+di/1 -> c_to_ri1/1(In1)
  c_to_ri1/1(Out1) -> cmult*/3(c)
  c_to_ri1/2(Out2) -> cmult*/4(d)
  acc_in/1 -> c_to_ri2/1(In1)
  acc/1(acc_out) -> ri_to_c/1(In1)
  acc1/1(acc_out) -> ri_to_c/2(In2)
  ri_to_c/1(Out1) -> acc_out/1
  c_to_ri2/1(Out1) -> acc/3(acc_in)
  c_to_ri2/2(Out2) -> acc1/3(acc_in)
  Relational/1 -> acc/1(rst), acc1/1(rst)
  Counter/1 -> Relational/1
  Constant1/1 -> Relational/2
  sync/1 -> Delay/1
  Delay/1 -> Counter/1
  Constant2/1 -> acc/4(valid_in)
  acc/2(valid_out) -> Terminator/1
  acc1/2(valid_out) -> valid_out/1
  valid_in/1 -> acc1/4(valid_in)

== system b_2x_8a_r308d/win_x_engine1/baseline_tap4/dual_pol_cmac/cmac2 ==
  a+bi : Inport  Port=1  LatchInput=off
  c+di : Inport  Port=2  LatchInput=off
  acc_in : Inport  Port=3  LatchInput=off
  sync : Inport  Port=4  LatchInput=off
  valid_in : Inport  Port=5  LatchInput=off
  Constant1 : xbsIndex_r3/Constant  const=0  equ=P=C  arith_type=Unsigned  n_bits=bit_growth  bin_pt=0  opselect=C  inp2=PCIN>>17  opr=+  inp1=P  carry=CIN  iostate=0  explicit_period=off  period=1  dbl_ovrd=off
  Constant2 : xbsIndex_r3/Constant  const=0  equ=P=C  arith_type=Unsigned  n_bits=1  bin_pt=0  opselect=C  inp2=PCIN>>17  opr=+  inp1=P  carry=CIN  iostate=0  explicit_period=off  period=1  dbl_ovrd=off
  Counter : xbsIndex_r3/Counter  cnt_type=Count Limited  n_bits=bit_growth  bin_pt=0  arith_type=Unsigned  start_count=0  cnt_to=acc_len - 1  cnt_by_val=1  operation=Up  explicit_period=off  period=1  load_pin=off  rst=on  en=off  dbl_ovrd=off  show_param=off  use_rpm=on  gen_core=off
      settings: xl_area=[0, 0, 0, 0, 0, 0, 0]
  Delay : xbsIndex_r3/Delay  latency=add_latency + mult_latency - 1  reg_retiming=off  explicit_period=off  period=1  en=off  accept_only_valid=off  init_zero=on  dbl_ovrd=off  show_param=off
      settings: xl_area=[0, 0, 0, 0, 0, 0, 0]
  Relational : xbsIndex_r3/Relational  mode=a=b  latency=1  explicit_period=off  period=1  en=off  dbl_ovrd=off  show_param=off
      settings: xl_area=[0, 0, 0, 0, 0, 0, 0]
  Terminator : Terminator
  acc : Subsystem
  acc1 : Subsystem
  c_to_ri : Subsystem
  c_to_ri1 : Subsystem
  c_to_ri2 : Subsystem
  cmult* : Subsystem  BlockChoice=cmult_4bit_em*
      link override cmult_4bit_br*: mult_latency=mult_latency  add_latency=add_latency
      link override cmult_4bit_em*: mult_latency=mult_latency  add_latency=add_latency
      link override cmult_4bit_sl*: mult_latency=mult_latency  add_latency=add_latency
      settings: AttributesFormatString=%<BlockChoice>  TemplateBlock=casper_library/Multipliers/cmult*  MemberBlocks=cmult_4bit_br*,cmult_4bit_em*,cmult_4bit_sl*
      mask Type: cmult*
  ri_to_c : Subsystem
  acc_out : Outport
  valid_out : Outport  Port=2
  wires:
  valid_in/1 -> acc1/4(valid_in)
  acc1/2(valid_out) -> valid_out/1
  acc/2(valid_out) -> Terminator/1
  Constant2/1 -> acc/4(valid_in)
  Delay/1 -> Counter/1
  sync/1 -> Delay/1
  Constant1/1 -> Relational/2
  Counter/1 -> Relational/1
  Relational/1 -> acc1/1(rst), acc/1(rst)
  c_to_ri2/2(Out2) -> acc1/3(acc_in)
  c_to_ri2/1(Out1) -> acc/3(acc_in)
  ri_to_c/1(Out1) -> acc_out/1
  acc1/1(acc_out) -> ri_to_c/2(In2)
  acc/1(acc_out) -> ri_to_c/1(In1)
  acc_in/1 -> c_to_ri2/1(In1)
  c_to_ri1/2(Out2) -> cmult*/4(d)
  c_to_ri1/1(Out1) -> cmult*/3(c)
  c+di/1 -> c_to_ri1/1(In1)
  c_to_ri/2(Out2) -> cmult*/2(b)
  c_to_ri/1(Out1) -> cmult*/1(a)
  a+bi/1 -> c_to_ri/1(In1)
  cmult*/2(imag) -> acc1/2(din)
  cmult*/1(real) -> acc/2(din)

== system b_2x_8a_r308d/win_x_engine1/baseline_tap4/dual_pol_cmac/cmac3 ==
  a+bi : Inport  Port=1  LatchInput=off
  c+di : Inport  Port=2  LatchInput=off
  acc_in : Inport  Port=3  LatchInput=off
  sync : Inport  Port=4  LatchInput=off
  valid_in : Inport  Port=5  LatchInput=off
  Constant1 : xbsIndex_r3/Constant  const=0  equ=P=C  arith_type=Unsigned  n_bits=bit_growth  bin_pt=0  opselect=C  inp2=PCIN>>17  opr=+  inp1=P  carry=CIN  iostate=0  explicit_period=off  period=1  dbl_ovrd=off
  Constant2 : xbsIndex_r3/Constant  const=0  equ=P=C  arith_type=Unsigned  n_bits=1  bin_pt=0  opselect=C  inp2=PCIN>>17  opr=+  inp1=P  carry=CIN  iostate=0  explicit_period=off  period=1  dbl_ovrd=off
  Counter : xbsIndex_r3/Counter  cnt_type=Count Limited  n_bits=bit_growth  bin_pt=0  arith_type=Unsigned  start_count=0  cnt_to=acc_len - 1  cnt_by_val=1  operation=Up  explicit_period=off  period=1  load_pin=off  rst=on  en=off  dbl_ovrd=off  show_param=off  use_rpm=on  gen_core=off
      settings: xl_area=[0, 0, 0, 0, 0, 0, 0]
  Delay : xbsIndex_r3/Delay  latency=add_latency + mult_latency - 1  reg_retiming=off  explicit_period=off  period=1  en=off  accept_only_valid=off  init_zero=on  dbl_ovrd=off  show_param=off
      settings: xl_area=[0, 0, 0, 0, 0, 0, 0]
  Relational : xbsIndex_r3/Relational  mode=a=b  latency=1  explicit_period=off  period=1  en=off  dbl_ovrd=off  show_param=off
      settings: xl_area=[0, 0, 0, 0, 0, 0, 0]
  Terminator : Terminator
  acc : Subsystem
  acc1 : Subsystem
  c_to_ri : Subsystem
  c_to_ri1 : Subsystem
  c_to_ri2 : Subsystem
  cmult* : Subsystem  BlockChoice=cmult_4bit_em*
      link override cmult_4bit_br*: mult_latency=mult_latency  add_latency=add_latency
      link override cmult_4bit_em*: mult_latency=mult_latency  add_latency=add_latency
      link override cmult_4bit_sl*: mult_latency=mult_latency  add_latency=add_latency
      settings: AttributesFormatString=%<BlockChoice>  TemplateBlock=casper_library/Multipliers/cmult*  MemberBlocks=cmult_4bit_br*,cmult_4bit_em*,cmult_4bit_sl*
      mask Type: cmult*
  ri_to_c : Subsystem
  acc_out : Outport
  valid_out : Outport  Port=2
  wires:
  valid_in/1 -> acc1/4(valid_in)
  acc1/2(valid_out) -> valid_out/1
  acc/2(valid_out) -> Terminator/1
  Constant2/1 -> acc/4(valid_in)
  Delay/1 -> Counter/1
  sync/1 -> Delay/1
  Constant1/1 -> Relational/2
  Counter/1 -> Relational/1
  Relational/1 -> acc1/1(rst), acc/1(rst)
  c_to_ri2/2(Out2) -> acc1/3(acc_in)
  c_to_ri2/1(Out1) -> acc/3(acc_in)
  ri_to_c/1(Out1) -> acc_out/1
  acc1/1(acc_out) -> ri_to_c/2(In2)
  acc/1(acc_out) -> ri_to_c/1(In1)
  acc_in/1 -> c_to_ri2/1(In1)
  c_to_ri1/2(Out2) -> cmult*/4(d)
  c_to_ri1/1(Out1) -> cmult*/3(c)
  c+di/1 -> c_to_ri1/1(In1)
  c_to_ri/2(Out2) -> cmult*/2(b)
  c_to_ri/1(Out1) -> cmult*/1(a)
  a+bi/1 -> c_to_ri/1(In1)
  cmult*/2(imag) -> acc1/2(din)
  cmult*/1(real) -> acc/2(din)

== system b_2x_8a_r308d/win_x_engine1/baseline_tap4/dual_pol_cmac/cmac4 ==
  a+bi : Inport  Port=1  LatchInput=off
  c+di : Inport  Port=2  LatchInput=off
  acc_in : Inport  Port=3  LatchInput=off
  sync : Inport  Port=4  LatchInput=off
  valid_in : Inport  Port=5  LatchInput=off
  Constant1 : xbsIndex_r3/Constant  const=0  equ=P=C  arith_type=Unsigned  n_bits=bit_growth  bin_pt=0  opselect=C  inp2=PCIN>>17  opr=+  inp1=P  carry=CIN  iostate=0  explicit_period=off  period=1  dbl_ovrd=off
  Constant2 : xbsIndex_r3/Constant  const=0  equ=P=C  arith_type=Unsigned  n_bits=1  bin_pt=0  opselect=C  inp2=PCIN>>17  opr=+  inp1=P  carry=CIN  iostate=0  explicit_period=off  period=1  dbl_ovrd=off
  Counter : xbsIndex_r3/Counter  cnt_type=Count Limited  n_bits=bit_growth  bin_pt=0  arith_type=Unsigned  start_count=0  cnt_to=acc_len - 1  cnt_by_val=1  operation=Up  explicit_period=off  period=1  load_pin=off  rst=on  en=off  dbl_ovrd=off  show_param=off  use_rpm=on  gen_core=off
      settings: xl_area=[0, 0, 0, 0, 0, 0, 0]
  Delay : xbsIndex_r3/Delay  latency=add_latency + mult_latency - 1  reg_retiming=off  explicit_period=off  period=1  en=off  accept_only_valid=off  init_zero=on  dbl_ovrd=off  show_param=off
      settings: xl_area=[0, 0, 0, 0, 0, 0, 0]
  Relational : xbsIndex_r3/Relational  mode=a=b  latency=1  explicit_period=off  period=1  en=off  dbl_ovrd=off  show_param=off
      settings: xl_area=[0, 0, 0, 0, 0, 0, 0]
  Terminator : Terminator
  acc : Subsystem
  acc1 : Subsystem
  c_to_ri : Subsystem
  c_to_ri1 : Subsystem
  c_to_ri2 : Subsystem
  cmult* : Subsystem  BlockChoice=cmult_4bit_em*
      link override cmult_4bit_br*: mult_latency=mult_latency  add_latency=add_latency
      link override cmult_4bit_em*: mult_latency=mult_latency  add_latency=add_latency
      link override cmult_4bit_sl*: mult_latency=mult_latency  add_latency=add_latency
      settings: AttributesFormatString=%<BlockChoice>  TemplateBlock=casper_library/Multipliers/cmult*  MemberBlocks=cmult_4bit_br*,cmult_4bit_em*,cmult_4bit_sl*
      mask Type: cmult*
  ri_to_c : Subsystem
  acc_out : Outport
  valid_out : Outport  Port=2
  wires:
  valid_in/1 -> acc1/4(valid_in)
  acc1/2(valid_out) -> valid_out/1
  acc/2(valid_out) -> Terminator/1
  Constant2/1 -> acc/4(valid_in)
  Delay/1 -> Counter/1
  sync/1 -> Delay/1
  Constant1/1 -> Relational/2
  Counter/1 -> Relational/1
  Relational/1 -> acc1/1(rst), acc/1(rst)
  c_to_ri2/2(Out2) -> acc1/3(acc_in)
  c_to_ri2/1(Out1) -> acc/3(acc_in)
  ri_to_c/1(Out1) -> acc_out/1
  acc1/1(acc_out) -> ri_to_c/2(In2)
  acc/1(acc_out) -> ri_to_c/1(In1)
  acc_in/1 -> c_to_ri2/1(In1)
  c_to_ri1/2(Out2) -> cmult*/4(d)
  c_to_ri1/1(Out1) -> cmult*/3(c)
  c+di/1 -> c_to_ri1/1(In1)
  c_to_ri/2(Out2) -> cmult*/2(b)
  c_to_ri/1(Out1) -> cmult*/1(a)
  a+bi/1 -> c_to_ri/1(In1)
  cmult*/2(imag) -> acc1/2(din)
  cmult*/1(real) -> acc/2(din)

== system b_2x_8a_r308d/win_x_engine1/x_engine_reorder/win1_ctrl/pulse_extender ==
  in : Inport  Port=1  LatchInput=off
  Constant : xbsIndex_r3/Constant  const=1  equ=P=C  arith_type=Boolean  n_bits=1  bin_pt=0  opselect=C  inp2=PCIN>>17  opr=+  inp1=P  carry=CIN  iostate=0  explicit_period=off  period=1  dbl_ovrd=off
  Constant17 : xbsIndex_r3/Constant  const=pulse_len  equ=P=C  arith_type=Unsigned  n_bits=bits  bin_pt=0  opselect=C  inp2=PCIN>>17  opr=+  inp1=P  carry=CIN  iostate=0  explicit_period=on  period=1  dbl_ovrd=off
  Inverter1 : xbsIndex_r3/Inverter  latency=0  explicit_period=off  period=1  en=off  dbl_ovrd=off  show_param=off
      settings: xl_area=[0, 0, 0, 0, 0, 0, 0]
  Logical2 : xbsIndex_r3/Logical  logical_function=AND  inputs=2  precision=Full  arith_type=Unsigned  n_bits=8  bin_pt=2  align_bp=on  latency=0  explicit_period=off  period=1  en=off  dbl_ovrd=off  show_param=off
      settings: xl_area=[0, 0, 0, 0, 0, 0, 0]
  Relational1 : xbsIndex_r3/Relational  mode=a<b  latency=0  explicit_period=off  period=1  en=off  dbl_ovrd=off  show_param=off
      settings: xl_area=[0, 0, 0, 0, 0, 0, 0]
  Slice : xbsIndex_r3/Slice  mode=Lower Bit Location + Width  nbits=1  bit1=0  base1=MSB of Input  bit0=0  base0=LSB of Input  boolean_output=on  explicit_period=off  period=1  dbl_ovrd=off
  Terminator : Terminator
  freeze_cntr : Subsystem  mask{CounterBits=bits}
      mask prompts: CounterBits "Counter Length (2^?)"
  posedge : Subsystem  Tag=Rising Edge Detector
  out : Outport
  wires:
  Inverter1/1 -> Logical2/1
  Slice/1 -> Inverter1/1
  Relational1/1 -> Logical2/2
  Logical2/1 -> out/1
  Constant/1 -> freeze_cntr/1(en)
  freeze_cntr/2(we) -> Terminator/1
  freeze_cntr/1(addr) -> Slice/1, Relational1/1
  posedge/1(Out) -> freeze_cntr/2(rst)
  Constant17/1 -> Relational1/2
  in/1 -> posedge/1(In)
